simulink model "bit4fulladddigital14"  (R2024a)
settings: Solver=VariableStepAuto  StartTime=0.0  StopTime=10.0  RelTol=1e-3
settings Model: Creator=vijit  LastModifiedBy=tusha
settings OptimizationCC: ReuseModelBlockBuffer=off
settings RTWCC: GPUComputeCapability=3.5

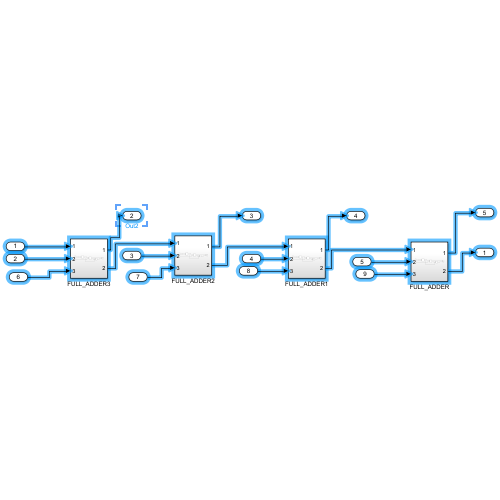
[thumbnail: Simulink's stored preview of the top-level diagram]
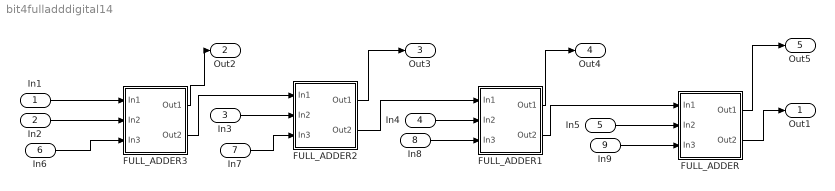
== system bit4fulladddigital14 ==
  In1 : Inport
  In2 : Inport  Port=2
  In3 : Inport  Port=3
  In4 : Inport  Port=4
  In5 : Inport  Port=5
  In6 : Inport  Port=6
  In7 : Inport  Port=7
  In8 : Inport  Port=8
  In9 : Inport  Port=9
  FULL_ADDER : Subsystem
  FULL_ADDER1 : Subsystem
  FULL_ADDER2 : Subsystem
  FULL_ADDER3 : Subsystem
  Out1 : Outport
  Out2 : Outport  Port=2
  Out3 : Outport  Port=3
  Out4 : Outport  Port=4
  Out5 : Outport  Port=5
  wires:
  In1/1 -> FULL_ADDER3/1(In1)
  In2/1 -> FULL_ADDER3/2(In2)
  In6/1 -> FULL_ADDER3/3(In3)
  FULL_ADDER3/2(Out2) -> FULL_ADDER2/1(In1)
  In3/1 -> FULL_ADDER2/2(In2)
  In7/1 -> FULL_ADDER2/3(In3)
  FULL_ADDER2/2(Out2) -> FULL_ADDER1/1(In1)
  In4/1 -> FULL_ADDER1/2(In2)
  In8/1 -> FULL_ADDER1/3(In3)
  FULL_ADDER1/2(Out2) -> FULL_ADDER/1(In1)
  In5/1 -> FULL_ADDER/2(In2)
  In9/1 -> FULL_ADDER/3(In3)
  FULL_ADDER/2(Out2) -> Out1/1
  FULL_ADDER3/1(Out1) -> Out2/1
  FULL_ADDER2/1(Out1) -> Out3/1
  FULL_ADDER1/1(Out1) -> Out4/1
  FULL_ADDER/1(Out1) -> Out5/1

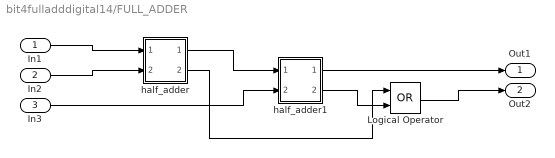
== system bit4fulladddigital14/FULL_ADDER ==
  In1 : Inport
  In2 : Inport  Port=2
  In3 : Inport  Port=3
  Logical Operator : Logic  Operator=OR  AllPortsSameDT=off  OutDataTypeStr=boolean
  half_adder : Subsystem
  half_adder1 : Subsystem
  Out1 : Outport
  Out2 : Outport  Port=2
  wires:
  half_adder1/2(Out2) -> Logical Operator/2
  In3/1 -> half_adder1/2(In2)
  In1/1 -> half_adder/1(In1)
  half_adder1/1(Out1) -> Out1/1
  half_adder/1(Out1) -> half_adder1/1(In1)
  half_adder/2(Out2) -> Logical Operator/1
  In2/1 -> half_adder/2(In2)
  Logical Operator/1 -> Out2/1

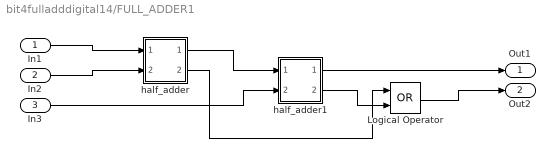
== system bit4fulladddigital14/FULL_ADDER1 ==
  In1 : Inport
  In2 : Inport  Port=2
  In3 : Inport  Port=3
  Logical Operator : Logic  Operator=OR  AllPortsSameDT=off  OutDataTypeStr=boolean
  half_adder : Subsystem
  half_adder1 : Subsystem
  Out1 : Outport
  Out2 : Outport  Port=2
  wires:
  half_adder1/2(Out2) -> Logical Operator/2
  In3/1 -> half_adder1/2(In2)
  In1/1 -> half_adder/1(In1)
  half_adder1/1(Out1) -> Out1/1
  half_adder/1(Out1) -> half_adder1/1(In1)
  half_adder/2(Out2) -> Logical Operator/1
  In2/1 -> half_adder/2(In2)
  Logical Operator/1 -> Out2/1

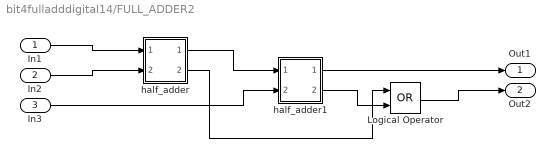
== system bit4fulladddigital14/FULL_ADDER2 ==
  In1 : Inport
  In2 : Inport  Port=2
  In3 : Inport  Port=3
  Logical Operator : Logic  Operator=OR  AllPortsSameDT=off  OutDataTypeStr=boolean
  half_adder : Subsystem
  half_adder1 : Subsystem
  Out1 : Outport
  Out2 : Outport  Port=2
  wires:
  half_adder1/2(Out2) -> Logical Operator/2
  In3/1 -> half_adder1/2(In2)
  In1/1 -> half_adder/1(In1)
  half_adder1/1(Out1) -> Out1/1
  half_adder/1(Out1) -> half_adder1/1(In1)
  half_adder/2(Out2) -> Logical Operator/1
  In2/1 -> half_adder/2(In2)
  Logical Operator/1 -> Out2/1

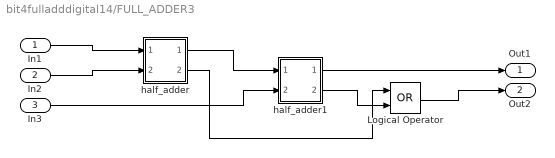
== system bit4fulladddigital14/FULL_ADDER3 ==
  In1 : Inport
  In2 : Inport  Port=2
  In3 : Inport  Port=3
  Logical Operator : Logic  Operator=OR  AllPortsSameDT=off  OutDataTypeStr=boolean
  half_adder : Subsystem
  half_adder1 : Subsystem
  Out1 : Outport
  Out2 : Outport  Port=2
  wires:
  half_adder1/2(Out2) -> Logical Operator/2
  In3/1 -> half_adder1/2(In2)
  In1/1 -> half_adder/1(In1)
  half_adder1/1(Out1) -> Out1/1
  half_adder/1(Out1) -> half_adder1/1(In1)
  half_adder/2(Out2) -> Logical Operator/1
  In2/1 -> half_adder/2(In2)
  Logical Operator/1 -> Out2/1

== system bit4fulladddigital14/FULL_ADDER/half_adder ==
  In1 : Inport
  In2 : Inport  Port=2
  Logical Operator1 : Logic  AllPortsSameDT=off  OutDataTypeStr=boolean
  XOR_BASIC : Subsystem
  Out1 : Outport
  Out2 : Outport  Port=2
  wires:
  In1/1 -> XOR_BASIC/1(In1), Logical Operator1/1
  In2/1 -> XOR_BASIC/2(In2), Logical Operator1/2
  Logical Operator1/1 -> Out2/1
  XOR_BASIC/1(Out1) -> Out1/1

== system bit4fulladddigital14/FULL_ADDER/half_adder1 ==
  In1 : Inport
  In2 : Inport  Port=2
  Logical Operator1 : Logic  AllPortsSameDT=off  OutDataTypeStr=boolean
  XOR_BASIC : Subsystem
  Out1 : Outport
  Out2 : Outport  Port=2
  wires:
  In1/1 -> XOR_BASIC/1(In1), Logical Operator1/1
  In2/1 -> XOR_BASIC/2(In2), Logical Operator1/2
  Logical Operator1/1 -> Out2/1
  XOR_BASIC/1(Out1) -> Out1/1

== system bit4fulladddigital14/FULL_ADDER1/half_adder ==
  In1 : Inport
  In2 : Inport  Port=2
  Logical Operator1 : Logic  AllPortsSameDT=off  OutDataTypeStr=boolean
  XOR_BASIC : Subsystem
  Out1 : Outport
  Out2 : Outport  Port=2
  wires:
  In1/1 -> XOR_BASIC/1(In1), Logical Operator1/1
  In2/1 -> XOR_BASIC/2(In2), Logical Operator1/2
  Logical Operator1/1 -> Out2/1
  XOR_BASIC/1(Out1) -> Out1/1

== system bit4fulladddigital14/FULL_ADDER1/half_adder1 ==
  In1 : Inport
  In2 : Inport  Port=2
  Logical Operator1 : Logic  AllPortsSameDT=off  OutDataTypeStr=boolean
  XOR_BASIC : Subsystem
  Out1 : Outport
  Out2 : Outport  Port=2
  wires:
  In1/1 -> XOR_BASIC/1(In1), Logical Operator1/1
  In2/1 -> XOR_BASIC/2(In2), Logical Operator1/2
  Logical Operator1/1 -> Out2/1
  XOR_BASIC/1(Out1) -> Out1/1

== system bit4fulladddigital14/FULL_ADDER2/half_adder ==
  In1 : Inport
  In2 : Inport  Port=2
  Logical Operator1 : Logic  AllPortsSameDT=off  OutDataTypeStr=boolean
  XOR_BASIC : Subsystem
  Out1 : Outport
  Out2 : Outport  Port=2
  wires:
  In1/1 -> XOR_BASIC/1(In1), Logical Operator1/1
  In2/1 -> XOR_BASIC/2(In2), Logical Operator1/2
  Logical Operator1/1 -> Out2/1
  XOR_BASIC/1(Out1) -> Out1/1

== system bit4fulladddigital14/FULL_ADDER2/half_adder1 ==
  In1 : Inport
  In2 : Inport  Port=2
  Logical Operator1 : Logic  AllPortsSameDT=off  OutDataTypeStr=boolean
  XOR_BASIC : Subsystem
  Out1 : Outport
  Out2 : Outport  Port=2
  wires:
  In1/1 -> XOR_BASIC/1(In1), Logical Operator1/1
  In2/1 -> XOR_BASIC/2(In2), Logical Operator1/2
  Logical Operator1/1 -> Out2/1
  XOR_BASIC/1(Out1) -> Out1/1

== system bit4fulladddigital14/FULL_ADDER3/half_adder ==
  In1 : Inport
  In2 : Inport  Port=2
  Logical Operator1 : Logic  AllPortsSameDT=off  OutDataTypeStr=boolean
  XOR_BASIC : Subsystem
  Out1 : Outport
  Out2 : Outport  Port=2
  wires:
  In1/1 -> XOR_BASIC/1(In1), Logical Operator1/1
  In2/1 -> XOR_BASIC/2(In2), Logical Operator1/2
  Logical Operator1/1 -> Out2/1
  XOR_BASIC/1(Out1) -> Out1/1

== system bit4fulladddigital14/FULL_ADDER3/half_adder1 ==
  In1 : Inport
  In2 : Inport  Port=2
  Logical Operator1 : Logic  AllPortsSameDT=off  OutDataTypeStr=boolean
  XOR_BASIC : Subsystem
  Out1 : Outport
  Out2 : Outport  Port=2
  wires:
  In1/1 -> XOR_BASIC/1(In1), Logical Operator1/1
  In2/1 -> XOR_BASIC/2(In2), Logical Operator1/2
  Logical Operator1/1 -> Out2/1
  XOR_BASIC/1(Out1) -> Out1/1

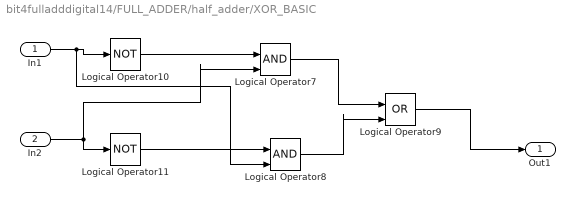
== system bit4fulladddigital14/FULL_ADDER/half_adder/XOR_BASIC ==
  In1 : Inport
  In2 : Inport  Port=2
  Logical Operator10 : Logic  Operator=NOT  IconShape=distinctive  AllPortsSameDT=off  OutDataTypeStr=boolean
  Logical Operator11 : Logic  Operator=NOT  IconShape=distinctive  AllPortsSameDT=off  OutDataTypeStr=boolean
  Logical Operator7 : Logic  IconShape=distinctive  AllPortsSameDT=off  OutDataTypeStr=boolean
  Logical Operator8 : Logic  IconShape=distinctive  AllPortsSameDT=off  OutDataTypeStr=boolean
  Logical Operator9 : Logic  Operator=OR  IconShape=distinctive  AllPortsSameDT=off  OutDataTypeStr=boolean
  Out1 : Outport
  wires:
  Logical Operator8/1 -> Logical Operator9/2
  Logical Operator7/1 -> Logical Operator9/1
  In2/1 -> Logical Operator7/2, Logical Operator11/1
  Logical Operator11/1 -> Logical Operator8/1
  Logical Operator9/1 -> Out1/1
  In1/1 -> Logical Operator8/2, Logical Operator10/1
  Logical Operator10/1 -> Logical Operator7/1

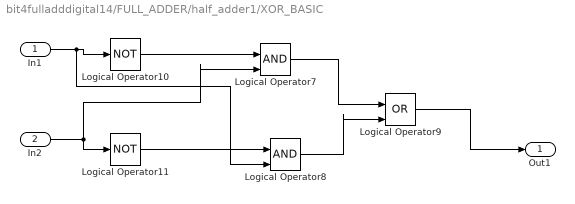
== system bit4fulladddigital14/FULL_ADDER/half_adder1/XOR_BASIC ==
  In1 : Inport
  In2 : Inport  Port=2
  Logical Operator10 : Logic  Operator=NOT  IconShape=distinctive  AllPortsSameDT=off  OutDataTypeStr=boolean
  Logical Operator11 : Logic  Operator=NOT  IconShape=distinctive  AllPortsSameDT=off  OutDataTypeStr=boolean
  Logical Operator7 : Logic  IconShape=distinctive  AllPortsSameDT=off  OutDataTypeStr=boolean
  Logical Operator8 : Logic  IconShape=distinctive  AllPortsSameDT=off  OutDataTypeStr=boolean
  Logical Operator9 : Logic  Operator=OR  IconShape=distinctive  AllPortsSameDT=off  OutDataTypeStr=boolean
  Out1 : Outport
  wires:
  Logical Operator8/1 -> Logical Operator9/2
  Logical Operator7/1 -> Logical Operator9/1
  In2/1 -> Logical Operator7/2, Logical Operator11/1
  Logical Operator11/1 -> Logical Operator8/1
  Logical Operator9/1 -> Out1/1
  In1/1 -> Logical Operator8/2, Logical Operator10/1
  Logical Operator10/1 -> Logical Operator7/1

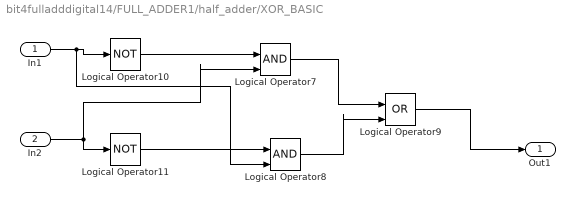
== system bit4fulladddigital14/FULL_ADDER1/half_adder/XOR_BASIC ==
  In1 : Inport
  In2 : Inport  Port=2
  Logical Operator10 : Logic  Operator=NOT  IconShape=distinctive  AllPortsSameDT=off  OutDataTypeStr=boolean
  Logical Operator11 : Logic  Operator=NOT  IconShape=distinctive  AllPortsSameDT=off  OutDataTypeStr=boolean
  Logical Operator7 : Logic  IconShape=distinctive  AllPortsSameDT=off  OutDataTypeStr=boolean
  Logical Operator8 : Logic  IconShape=distinctive  AllPortsSameDT=off  OutDataTypeStr=boolean
  Logical Operator9 : Logic  Operator=OR  IconShape=distinctive  AllPortsSameDT=off  OutDataTypeStr=boolean
  Out1 : Outport
  wires:
  Logical Operator8/1 -> Logical Operator9/2
  Logical Operator7/1 -> Logical Operator9/1
  In2/1 -> Logical Operator7/2, Logical Operator11/1
  Logical Operator11/1 -> Logical Operator8/1
  Logical Operator9/1 -> Out1/1
  In1/1 -> Logical Operator8/2, Logical Operator10/1
  Logical Operator10/1 -> Logical Operator7/1

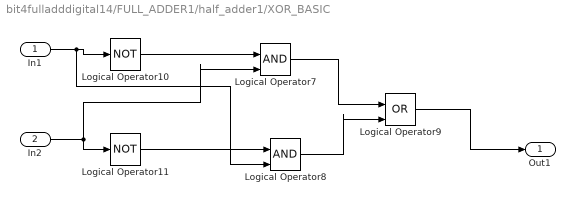
== system bit4fulladddigital14/FULL_ADDER1/half_adder1/XOR_BASIC ==
  In1 : Inport
  In2 : Inport  Port=2
  Logical Operator10 : Logic  Operator=NOT  IconShape=distinctive  AllPortsSameDT=off  OutDataTypeStr=boolean
  Logical Operator11 : Logic  Operator=NOT  IconShape=distinctive  AllPortsSameDT=off  OutDataTypeStr=boolean
  Logical Operator7 : Logic  IconShape=distinctive  AllPortsSameDT=off  OutDataTypeStr=boolean
  Logical Operator8 : Logic  IconShape=distinctive  AllPortsSameDT=off  OutDataTypeStr=boolean
  Logical Operator9 : Logic  Operator=OR  IconShape=distinctive  AllPortsSameDT=off  OutDataTypeStr=boolean
  Out1 : Outport
  wires:
  Logical Operator8/1 -> Logical Operator9/2
  Logical Operator7/1 -> Logical Operator9/1
  In2/1 -> Logical Operator7/2, Logical Operator11/1
  Logical Operator11/1 -> Logical Operator8/1
  Logical Operator9/1 -> Out1/1
  In1/1 -> Logical Operator8/2, Logical Operator10/1
  Logical Operator10/1 -> Logical Operator7/1

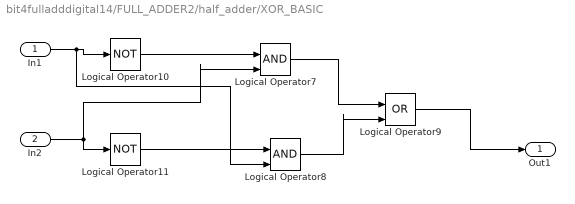
== system bit4fulladddigital14/FULL_ADDER2/half_adder/XOR_BASIC ==
  In1 : Inport
  In2 : Inport  Port=2
  Logical Operator10 : Logic  Operator=NOT  IconShape=distinctive  AllPortsSameDT=off  OutDataTypeStr=boolean
  Logical Operator11 : Logic  Operator=NOT  IconShape=distinctive  AllPortsSameDT=off  OutDataTypeStr=boolean
  Logical Operator7 : Logic  IconShape=distinctive  AllPortsSameDT=off  OutDataTypeStr=boolean
  Logical Operator8 : Logic  IconShape=distinctive  AllPortsSameDT=off  OutDataTypeStr=boolean
  Logical Operator9 : Logic  Operator=OR  IconShape=distinctive  AllPortsSameDT=off  OutDataTypeStr=boolean
  Out1 : Outport
  wires:
  Logical Operator8/1 -> Logical Operator9/2
  Logical Operator7/1 -> Logical Operator9/1
  In2/1 -> Logical Operator7/2, Logical Operator11/1
  Logical Operator11/1 -> Logical Operator8/1
  Logical Operator9/1 -> Out1/1
  In1/1 -> Logical Operator8/2, Logical Operator10/1
  Logical Operator10/1 -> Logical Operator7/1

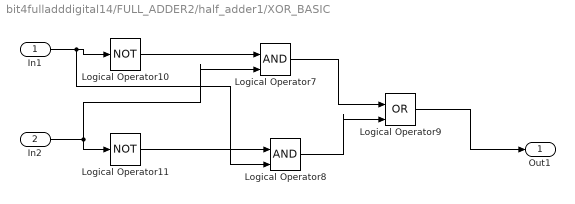
== system bit4fulladddigital14/FULL_ADDER2/half_adder1/XOR_BASIC ==
  In1 : Inport
  In2 : Inport  Port=2
  Logical Operator10 : Logic  Operator=NOT  IconShape=distinctive  AllPortsSameDT=off  OutDataTypeStr=boolean
  Logical Operator11 : Logic  Operator=NOT  IconShape=distinctive  AllPortsSameDT=off  OutDataTypeStr=boolean
  Logical Operator7 : Logic  IconShape=distinctive  AllPortsSameDT=off  OutDataTypeStr=boolean
  Logical Operator8 : Logic  IconShape=distinctive  AllPortsSameDT=off  OutDataTypeStr=boolean
  Logical Operator9 : Logic  Operator=OR  IconShape=distinctive  AllPortsSameDT=off  OutDataTypeStr=boolean
  Out1 : Outport
  wires:
  Logical Operator8/1 -> Logical Operator9/2
  Logical Operator7/1 -> Logical Operator9/1
  In2/1 -> Logical Operator7/2, Logical Operator11/1
  Logical Operator11/1 -> Logical Operator8/1
  Logical Operator9/1 -> Out1/1
  In1/1 -> Logical Operator8/2, Logical Operator10/1
  Logical Operator10/1 -> Logical Operator7/1

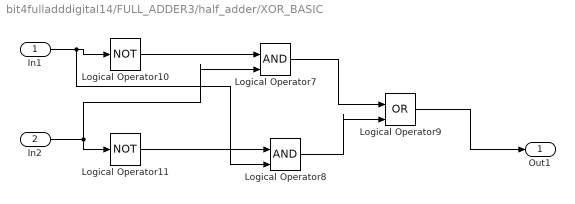
== system bit4fulladddigital14/FULL_ADDER3/half_adder/XOR_BASIC ==
  In1 : Inport
  In2 : Inport  Port=2
  Logical Operator10 : Logic  Operator=NOT  IconShape=distinctive  AllPortsSameDT=off  OutDataTypeStr=boolean
  Logical Operator11 : Logic  Operator=NOT  IconShape=distinctive  AllPortsSameDT=off  OutDataTypeStr=boolean
  Logical Operator7 : Logic  IconShape=distinctive  AllPortsSameDT=off  OutDataTypeStr=boolean
  Logical Operator8 : Logic  IconShape=distinctive  AllPortsSameDT=off  OutDataTypeStr=boolean
  Logical Operator9 : Logic  Operator=OR  IconShape=distinctive  AllPortsSameDT=off  OutDataTypeStr=boolean
  Out1 : Outport
  wires:
  Logical Operator8/1 -> Logical Operator9/2
  Logical Operator7/1 -> Logical Operator9/1
  In2/1 -> Logical Operator7/2, Logical Operator11/1
  Logical Operator11/1 -> Logical Operator8/1
  Logical Operator9/1 -> Out1/1
  In1/1 -> Logical Operator8/2, Logical Operator10/1
  Logical Operator10/1 -> Logical Operator7/1

== system bit4fulladddigital14/FULL_ADDER3/half_adder1/XOR_BASIC ==
  In1 : Inport
  In2 : Inport  Port=2
  Logical Operator10 : Logic  Operator=NOT  IconShape=distinctive  AllPortsSameDT=off  OutDataTypeStr=boolean
  Logical Operator11 : Logic  Operator=NOT  IconShape=distinctive  AllPortsSameDT=off  OutDataTypeStr=boolean
  Logical Operator7 : Logic  IconShape=distinctive  AllPortsSameDT=off  OutDataTypeStr=boolean
  Logical Operator8 : Logic  IconShape=distinctive  AllPortsSameDT=off  OutDataTypeStr=boolean
  Logical Operator9 : Logic  Operator=OR  IconShape=distinctive  AllPortsSameDT=off  OutDataTypeStr=boolean
  Out1 : Outport
  wires:
  Logical Operator8/1 -> Logical Operator9/2
  Logical Operator7/1 -> Logical Operator9/1
  In2/1 -> Logical Operator7/2, Logical Operator11/1
  Logical Operator11/1 -> Logical Operator8/1
  Logical Operator9/1 -> Out1/1
  In1/1 -> Logical Operator8/2, Logical Operator10/1
  Logical Operator10/1 -> Logical Operator7/1
